simulink model "speed"  (R2016b)
settings: Solver=VariableStepAuto  StartTime=0.0  StopTime=20  RelTol=1e-3
settings Model: Creator=nguyenquoctruong  LastModifiedBy=nguyenquoctruong

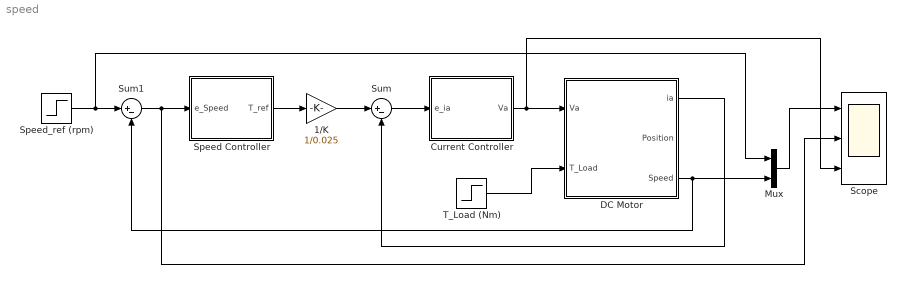
== system speed ==
  1/K : Gain  Gain=1/0.025
  Current Controller : Subsystem  mask{Kp=0.5, Ki=0.1, Vmax=12}
      mask prompts: Vmax "Vmax(V)"
  DC Motor : Subsystem  mask{Ra=0.1, K=0.025, Ja=0.0025, La=2*(10^-3), b=0.0002}
      mask prompts: Ra "Ra(Ohm)"; K "K(Vs)"; Ja "Ja(kgm^2)"; La "La(H)"; b "b(Nm.s.rad^-1)"
  Mux : Mux  Inputs=2
  Scope : Scope  NumInputPorts=3
  Speed Controller : Subsystem  mask{Kp=3, Ki=0.01, Tmax=2.66}
      mask prompts: Tmax "Tmax(Nm)"
  Speed_ref (rpm) : Step  Time=2.2  After=3000  SampleTime=0
  Sum : Sum  Inputs=|+-
  Sum1 : Sum  Inputs=|+-
  T_Load (Nm) : Step  Time=12  After=0.5  SampleTime=0
  wires:
  DC Motor/1(ia) -> Sum/2
  Sum1/1 -> Speed Controller/1(e_Speed), Scope/2
  Mux/1 -> Scope/1
  1/K/1 -> Sum/1
  Current Controller/1("Va ") -> DC Motor/1("Va "), Scope/3
  Sum/1 -> Current Controller/1(e_ia)
  Speed Controller/1("T_ref ") -> 1/K/1
  Speed_ref (rpm)/1 -> Mux/1, Sum1/1
  DC Motor/3("Speed ") -> Mux/2, Sum1/2
  T_Load (Nm)/1 -> DC Motor/2(T_Load)

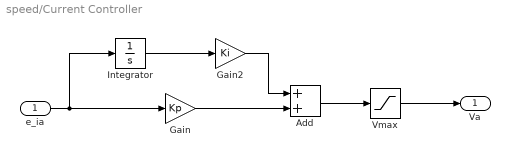
== system speed/Current Controller ==
  e_ia : Inport
  Add : Sum
  Gain : Gain  Gain=Kp
  Gain2 : Gain  Gain=Ki
  Integrator : Integrator
  Vmax : Saturate  UpperLimit=Vmax  LowerLimit=-Vmax
  "Va " : Outport
  wires:
  Integrator/1 -> Gain2/1
  e_ia/1 -> Integrator/1, Gain/1
  Gain2/1 -> Add/1
  Add/1 -> Vmax/1
  Vmax/1 -> "Va "/1
  Gain/1 -> Add/2

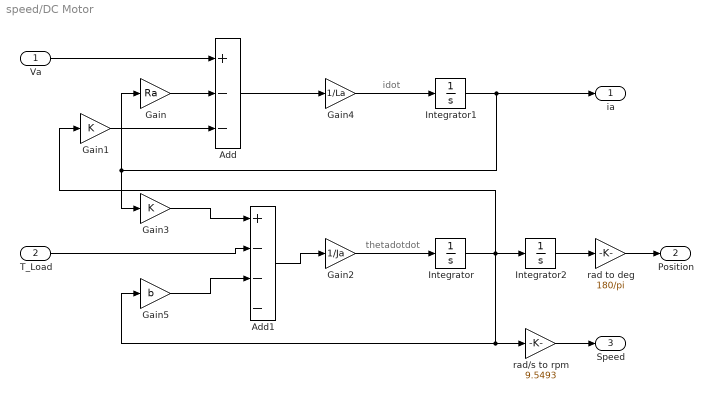
== system speed/DC Motor ==
  note: thetadotdot
  note: idot
  "Va " : Inport
  T_Load : Inport  Port=2
  Add : Sum  Inputs=+--
  Add1 : Sum  Inputs=+---
  Gain : Gain  Gain=Ra
  Gain1 : Gain  Gain=K
  Gain2 : Gain  Gain=1/Ja
  Gain3 : Gain  Gain=K
  Gain4 : Gain  Gain=1/La
  Gain5 : Gain  Gain=b
  Integrator : Integrator
  Integrator1 : Integrator
  Integrator2 : Integrator
  rad to deg : Gain  Gain=180/pi
  rad/s to rpm : Gain  Gain=9.5493
  ia : Outport
  Position : Outport  Port=2
  "Speed " : Outport  Port=3
  wires:
  Gain/1 -> Add/2
  T_Load/1 -> Add1/2
  Gain1/1 -> Add/3
  Gain3/1 -> Add1/1
  "Va "/1 -> Add/1
  Gain4/1 -> Integrator1/1
  Add/1 -> Gain4/1
  Add1/1 -> Gain2/1
  Gain2/1 -> Integrator/1
  Integrator1/1 -> ia/1, Gain/1, Gain3/1
  Integrator/1 -> Gain1/1, Integrator2/1, Gain5/1, rad/s to rpm/1
  Gain5/1 -> Add1/3
  rad/s to rpm/1 -> "Speed "/1
  Integrator2/1 -> rad to deg/1
  rad to deg/1 -> Position/1

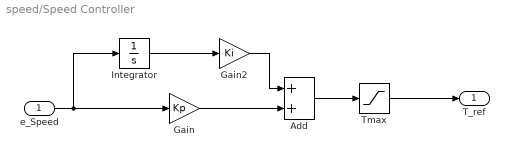
== system speed/Speed Controller ==
  e_Speed : Inport
  Add : Sum
  Gain : Gain  Gain=Kp
  Gain2 : Gain  Gain=Ki
  Integrator : Integrator
  Tmax : Saturate  UpperLimit=Tmax  LowerLimit=-Tmax
  "T_ref " : Outport
  wires:
  Tmax/1 -> "T_ref "/1
  Add/1 -> Tmax/1
  Gain2/1 -> Add/1
  Gain/1 -> Add/2
  e_Speed/1 -> Gain/1, Integrator/1
  Integrator/1 -> Gain2/1
